simulink model "chap6_1sim"  (Simulink 8.3)
settings: Solver=ode45  StartTime=0.0  StopTime=10.0  RelTol=1e-3
settings Model: Creator=AnTienPham  LastModifiedBy=AnTienPham
settings DataIOCC: SignalLoggingSaveFormat=Dataset
settings DebuggingCC: UnderspecifiedInitializationDetection=Simplified  StateNameClashWarn=none
settings GRTTargetCC: CombineOutputUpdateFcns=on  GRTInterface=off

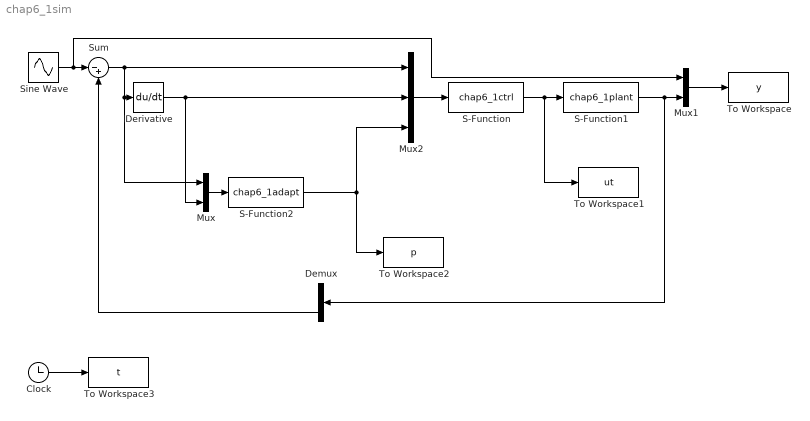
== system chap6_1sim ==
  Clock : Clock
  Demux : Demux  Outputs=2
  Derivative : Derivative
  Mux : Mux  Inputs=2
  Mux1 : Mux  Inputs=2
  Mux2 : Mux  Inputs=3
  S-Function : S-Function  FunctionName=chap6_1ctrl  EnableBusSupport=off
  S-Function1 : S-Function  FunctionName=chap6_1plant  EnableBusSupport=off
  S-Function2 : S-Function  FunctionName=chap6_1adapt  EnableBusSupport=off
  Sine Wave : Sin  SampleTime=0
  Sum : Sum  Inputs=|-+
  To Workspace : ToWorkspace  VariableName=y  SaveFormat=Timeseries  SampleTime=-1
  To Workspace1 : ToWorkspace  VariableName=ut  SaveFormat=Timeseries  SampleTime=-1
  To Workspace2 : ToWorkspace  VariableName=p  SaveFormat=Timeseries  SampleTime=-1
  To Workspace3 : ToWorkspace  VariableName=t  SaveFormat=Timeseries  SampleTime=-1
  wires:
  Sine Wave/1 -> Mux1/1, Sum/1
  Sum/1 -> Mux/1, Derivative/1, Mux2/1
  Derivative/1 -> Mux/2, Mux2/2
  Mux/1 -> S-Function2/1
  S-Function2/1 -> To Workspace2/1, Mux2/3
  S-Function/1 -> To Workspace1/1, S-Function1/1
  S-Function1/1 -> Demux/1, Mux1/2
  Mux1/1 -> To Workspace/1
  Demux/2 -> Sum/2
  Clock/1 -> To Workspace3/1
  Mux2/1 -> S-Function/1
